simulink model "Batteric_Pack"  (R2016a)
settings: Solver=VariableStepAuto  StartTime=0.0  StopTime=3600  RelTol=1e-3
undefined symbols (not defined in the file): Ion, Lithium
libraries: electricdrivelib x24, powerlib x4
settings Model: Creator=hp  LastModifiedBy=hp

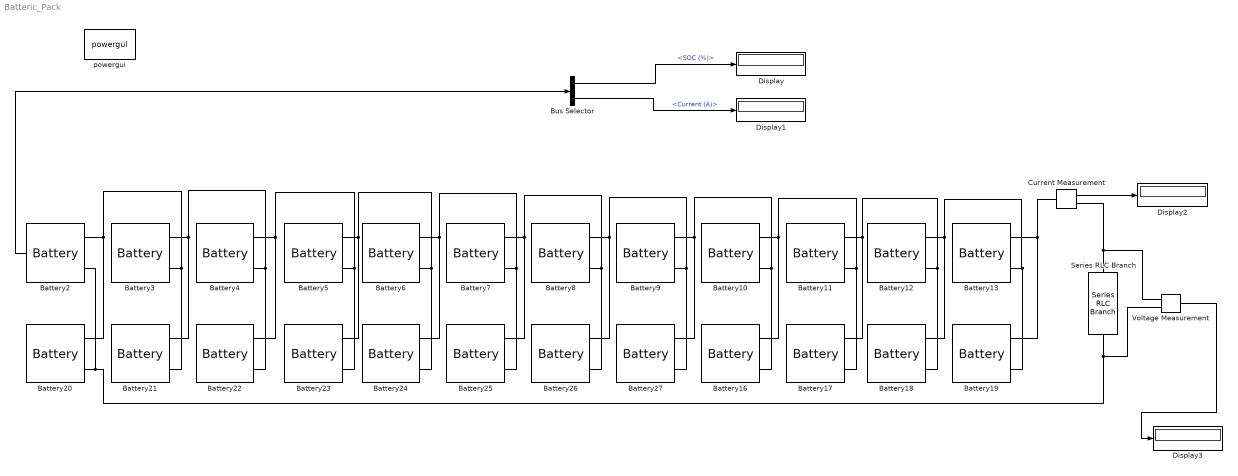
== system Batteric_Pack ==
  Battery{2..13,16..27} (24 alike) : electricdrivelib/Extra Sources/Battery  BatType=Lithium-Ion  ShowTempParam=off  ThermalPreset=no  NomV=3.7  NomQ=12.5  SOC=100  Batt_Tr=30  PresetModel=on  MaxQ=12.5  MinV=2.775  FullV=4.3068  Dis_rate=5.4348  R=0.00296  Normal_OP=11.3043  expZone="[3.9974     0.61413]"  current=[6.5 13 32.5]  Units=Time  Tci=20  NomT=25  T2=0  MaxQ2=2.208  FullV2=3.45  Normal_OP2=2.8  expZone2="[3.22        0.23]"  Rca=0.6  ti=1000  Dp=0
  Bus Selector : BusSelector  OutputSignals=SOC (%),Current (A)
  Current Measurement : powerlib/Measurements/Current Measurement  PhasorSimulation=off  OutputType=Complex  PSBequivalent=0
  Display{,1..3} (4 alike) : Display
  Series RLC Branch : powerlib/Elements/Series RLC Branch  LConnTagsString=__new0  RConnTagsString=__new0  BranchType=R  Resistance=3.55  Inductance=1e-3  SetiL0=off  InitialCurrent=0  Capacitance=1e-6  Setx0=off  InitialVoltage=0  Measurements=None
  Voltage Measurement : powerlib/Measurements/Voltage Measurement  PhasorSimulation=off  OutputType=Complex  PSBequivalent=0
  powergui : powerlib/powergui  Priority=1  SimulationMode=Continuous  SolverType=Tustin/Backward Euler (TBE)  SampleTime=50e-6  frequency=60  SPID=off  DisableSnubberDevices=off  DisableRonSwitches=off  DisableVfSwitches=off  SwTol=0  DisplayEquations=off  Interpol=off  ExternalGateDelay=off  methode=off  Ts=10  FunctionMessages=off  echomessages=off  HookPort=off  EnableUseOfTLC=off  x0status=blocks  frequencyindice=0  Pbase=100e6  ErrMax=1e-4  Iterations=50  UnitsV=kV  UnitsW=MW  buscounter=0  RestoreLinks=warning  ResistiveCurrentMeasurement=off  Frange=[0:2:500]  Ylog=off  Xlog=on  ShowGrid=off  save=off  variable=ZData  structure=0  ZoomFFT=off  StartTime=0.0  cycles=1  DisplayStyle=1  fundamental=60  FreqAxis=off  MaxFrequency=1000  frequencyindicesteady=1  RmsSteady=1  display=off
  wires:
  Battery2/1 -> Bus Selector/1
  Bus Selector/1 -> Display/1  "<SOC (%)>"
  Bus Selector/2 -> Display1/1  "<Current (A)>"
  Voltage Measurement/1 -> Display3/1
  Current Measurement/1 -> Display2/1
  connections:
  Battery20/LConn2 -- Voltage Measurement/LConn2 -- Series RLC Branch/RConn1 -- Battery2/LConn2
  Battery3/LConn1 -- Battery21/LConn1 -- Battery22/LConn2 -- Battery4/LConn2
  Battery4/LConn1 -- Battery22/LConn1 -- Battery23/LConn2 -- Battery5/LConn2
  Battery5/LConn1 -- Battery23/LConn1 -- Battery24/LConn2 -- Battery6/LConn2
  Battery6/LConn1 -- Battery24/LConn1 -- Battery25/LConn2 -- Battery7/LConn2
  Battery7/LConn1 -- Battery25/LConn1 -- Battery26/LConn2 -- Battery8/LConn2
  Battery8/LConn1 -- Battery26/LConn1 -- Battery27/LConn2 -- Battery9/LConn2
  Battery9/LConn1 -- Battery27/LConn1 -- Battery16/LConn2 -- Battery10/LConn2
  Battery10/LConn1 -- Battery16/LConn1 -- Battery17/LConn2 -- Battery11/LConn2
  Battery11/LConn1 -- Battery17/LConn1 -- Battery18/LConn2 -- Battery12/LConn2
  Battery12/LConn1 -- Battery18/LConn1 -- Battery19/LConn2 -- Battery13/LConn2
  Battery13/LConn1 -- Current Measurement/LConn1 -- Battery19/LConn1
  Battery2/LConn1 -- Battery20/LConn1 -- Battery21/LConn2 -- Battery3/LConn2
  Current Measurement/RConn1 -- Voltage Measurement/LConn1 -- Series RLC Branch/LConn1
